simulink model "Excavator_Mevea_BucketDriveline"  (R2026a)
settings: Solver=ode23t  StopTime=29.5  FixedStep=1e-5  MaxStep=Ts  AbsTol=1e-3
PostLoadFcn:
  | set_param(bdroot,'IgnoredZcDiagnostic','none');
  | Excavator_Test_Scenario_Select('loadedBucketDigCycle');
  | Excavator_Mevea_params
StartFcn:
  | tic
StopFcn:
  | elapsedSimTime = toc;
  | disp(['Elapsed Sim Time = ' num2str(elapsedSimTime)]);
model workspace: external: MAT-File ExcavatorAssemblyDataStruct.mat (data not in the file)
undefined symbols (not defined in the file or in its folder): AToBRegOrificeVector, AToTOrificeVector, BiPOrificeVector, BoomC, boomHEArea, boomREArea, boomUpMaxQ, boomValve, BToTOrificeVector, BucketC, bucketCloseMaxQ, bucketOpenMaxQ, BucketR, bucketValve, DiscIntNeverNeededParam, fluids, gravity, K, Lambda, LeftBoomR, maxPumpDisp, minPumpDisp, nominalEngineSpeed, P28Assembly, PToAOrificeVector, PToBOrificeVector, pumpCmdNegRateLimit, pumpCmdPosRateLimit, RightBoomR, StickC, stickInMaxQ, stickOutMaxQ, StickR, stickValve, SwingC, swingDisplacement, swingHighSpeedThreshold, swingMaxQ, SwingR, swingSpeedQGain, swingValve, tau, valveCmdNegRateLimit, valveCmdPosRateLimit, X, x0, Y, Z
libraries: fl_lib x113, SimscapeFluids_lib x78, nesl_utility x61, sm_lib x55, simulink_extras x11, Excavator_Parts_Lib x6, sm_wheel_loader_lib x6, simulink x5, sdl_lib x4, SignalEditorBlockLib x1
(part 2 of 8)

== system Excavator_Mevea_BucketDriveline/Excavator/Hydraulics/RightPump ==
  Cmd : Inport
  Mechanical Rotational Reference : fl_lib/Mechanical/Rotational Elements/Mechanical Rotational Reference
  PS-Simulink Converter2 : nesl_utility/PS-Simulink Converter  PhysicalDomain=network_engine_domain  SubClassName=ps_output  LeftPortType=input  RightPortType=output  PseudoPeriodic=off  Frequencies=[]  VectorFormat=1-D array  Unit=bar  AffineConversion=off
  RightPump : SimscapeFluids_lib/Isothermal Liquid/Pumps & Motors/Variable-Displacement Pump (IL)  leakage_friction_spec=fluids.isothermal_liquid.pumps_motors.enum.pump_motor_loss_spec.input_efficiency  displacement_nominal=30 cm^3/rev  omega_nominal=188 rad/s  p_nominal=10 MPa  vol_eff_nominal=0.92  mech_eff_nominal=0.88  no_load_torque=0 N*m  p_diff_eff_TLU=[.1, 1, 2] MPa  omega_eff_TLU=[25, 50, 100, 200, 300, 400] rad/s  displacement_eff_TLU=[-30, -19, 19, 30] cm^3/rev  vol_eff_TLU=repmat([.816, .908, .954, .977, .981, .984; .325, .663, .831, .916, .925, .946; .137, .568, .78, .892, .893, .91], 1, 1, 4)  mech_eff_TLU=repmat([.996, .996, .996, .996, .996, .996; .988, .989, .989, .989, .989, .99; .981, .981, .982, .982, .983, .984], 1, 1, 4)  p_diff_loss_TLU=[.1, 1, 2] MPa  omega_loss_TLU=[25, 50, 100, 200, 300, 400] rad/s  displacement_loss_TLU=[-30, -19, 19, 30] cm^3/rev  vol_loss_TLU=repmat(1e-3 * [.023, .023, .023, .023, .0285, .032; .0844, .0842, .0845, .084, .1125, .108; .1079, .108, .11, .108, .1605, .18], 1, 1, 4) m^3/s  mech_loss_TLU=repmat([.002, .002, .002, .002, .002, .002; .0607, .0556, .0556, .0556, .0556, .0505; .1937, .1937, .1833, .1833, .1729, .1626], 1, 1, 4) N*m  vol_eff_min=1e-3  vol_eff_max=1  mech_eff_min=1e-3  mech_eff_max=1  pressure_threshold=1e-3 MPa  omega_threshold=10 rad/s  displacement_threshold=0.1 cm^3/rev  supplied_range_check=simscape.enum.assert.action.none  pump_mode_check=simscape.enum.assert.action.none  pressure_check=simscape.enum.assert.action.none  p_min_valid=0.101325 MPa
  RightPumpEM : fl_lib/Physical Signals/Sources/PS Constant  constant=1
  RightPumpEV : fl_lib/Physical Signals/Sources/PS Constant  constant=1
  RightPumpPrSensor : fl_lib/Isothermal Liquid/Sensors/Pressure Sensor (IL)  pressure_measure=foundation.enum.pressure_measure.gauge
  RightPumpVolChamber : fl_lib/Isothermal Liquid/Elements/Constant Volume Chamber (IL)  volume=pumpChamberVol mm^3  p_I_specify=on  p_I_priority=High  p_I=p0 bar  p_I_nominal_specify=off  p_I_nominal_value=1  p_I_nominal_unit=MPa
  Simulink-PS Converter1 : nesl_utility/Simulink-PS Converter  PhysicalDomain=network_engine_domain  SubClassName=ps_input  LeftPortType=input  RightPortType=output  PseudoPeriodic=off  Frequencies=[]  NoiseDistribution=none  NoiseParameters=[]  Unit=cm^3/rev  AffineConversion=off  FilteringAndDerivatives=provide  SimscapeFilterOrder=1  InputFilterTimeConstant=0.001  UdotUserProvided=0
  Transfer Fcn (with initial outputs) : simulink_extras/Additional Linear/Transfer Fcn (with initial outputs)  N=[1]  D="[0.01  1]"  Y0=p0  U0=p0
  R : PMIOPort  Side=Left
  A : PMIOPort  Port=2  Side=Left
  B : PMIOPort  Port=3  Side=Right
  p : Outport
  wires:
  PS-Simulink Converter2/1 -> Transfer Fcn (with initial outputs)/1
  Transfer Fcn (with initial outputs)/1 -> p/1
  Cmd/1 -> Simulink-PS Converter1/1
  connections:
  RightPumpEV/RConn1 -- RightPump/LConn2
  RightPumpPrSensor/RConn1 -- PS-Simulink Converter2/LConn1
  B/RConn1 -- RightPump/LConn4 -- RightPumpPrSensor/LConn1 -- RightPumpVolChamber/LConn1
  Simulink-PS Converter1/RConn1 -- RightPump/LConn1
  RightPumpEM/RConn1 -- RightPump/LConn3
  R/RConn1 -- RightPump/RConn1
  RightPump/RConn3 -- A/RConn1
  RightPump/RConn2 -- Mechanical Rotational Reference/LConn1

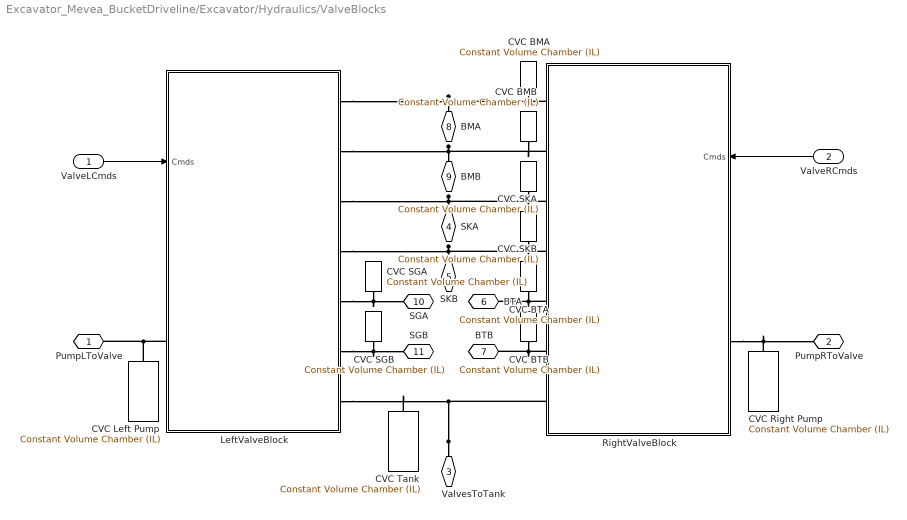
== system Excavator_Mevea_BucketDriveline/Excavator/Hydraulics/ValveBlocks ==
  ValveLCmds : Inport
  ValveRCmds : Inport  Port=2
  CVC BMA : fl_lib/Isothermal Liquid/Elements/Constant Volume Chamber (IL)  volume=vcVol m^3  p_I_specify=on  p_I_priority=High  p_I=initBoomHEPr bar  p_I_nominal_specify=off  p_I_nominal_value=1  p_I_nominal_unit=MPa
  CVC BMB : fl_lib/Isothermal Liquid/Elements/Constant Volume Chamber (IL)  volume=vcVol m^3  p_I_specify=on  p_I_priority=High  p_I=initBoomREPr bar  p_I_nominal_specify=off  p_I_nominal_value=1  p_I_nominal_unit=MPa
  CVC BTA : fl_lib/Isothermal Liquid/Elements/Constant Volume Chamber (IL)  volume=vcVol m^3  p_I_specify=on  p_I_priority=High  p_I=initBucketHEPr bar  p_I_nominal_specify=off  p_I_nominal_value=1  p_I_nominal_unit=MPa
  CVC BTB : fl_lib/Isothermal Liquid/Elements/Constant Volume Chamber (IL)  volume=vcVol m^3  p_I_specify=on  p_I_priority=High  p_I=initBucketREPr bar  p_I_nominal_specify=off  p_I_nominal_value=1  p_I_nominal_unit=MPa
  CVC Left Pump : fl_lib/Isothermal Liquid/Elements/Constant Volume Chamber (IL)  volume=vcVol m^3  p_I_specify=on  p_I_priority=High  p_I=p0 bar  p_I_nominal_specify=off  p_I_nominal_value=1  p_I_nominal_unit=MPa
  CVC Right Pump : fl_lib/Isothermal Liquid/Elements/Constant Volume Chamber (IL)  volume=vcVol m^3  p_I_specify=on  p_I_priority=High  p_I=p0 bar  p_I_nominal_specify=off  p_I_nominal_value=1  p_I_nominal_unit=MPa
  CVC SGA : fl_lib/Isothermal Liquid/Elements/Constant Volume Chamber (IL)  volume=vcVol m^3  p_I_specify=on  p_I_priority=High  p_I=initSwingAPr bar  p_I_nominal_specify=off  p_I_nominal_value=1  p_I_nominal_unit=MPa
  CVC SGB : fl_lib/Isothermal Liquid/Elements/Constant Volume Chamber (IL)  volume=vcVol m^3  p_I_specify=on  p_I_priority=High  p_I=initSwingBPr bar  p_I_nominal_specify=off  p_I_nominal_value=1  p_I_nominal_unit=MPa
  CVC SKA : fl_lib/Isothermal Liquid/Elements/Constant Volume Chamber (IL)  volume=vcVol m^3  p_I_specify=on  p_I_priority=High  p_I=initStickHEPr bar  p_I_nominal_specify=off  p_I_nominal_value=1  p_I_nominal_unit=MPa
  CVC SKB : fl_lib/Isothermal Liquid/Elements/Constant Volume Chamber (IL)  volume=vcVol m^3  p_I_specify=on  p_I_priority=High  p_I=initStickREPr bar  p_I_nominal_specify=off  p_I_nominal_value=1  p_I_nominal_unit=MPa
  CVC Tank : fl_lib/Isothermal Liquid/Elements/Constant Volume Chamber (IL)  volume=vcVol m^3  p_I_specify=off  p_I_priority=High  p_I=0.101325 MPa  p_I_nominal_specify=off  p_I_nominal_value=1  p_I_nominal_unit=MPa
  LeftValveBlock : Subsystem
      mask Display: image('Valve_Block_IMAGE.png');
  RightValveBlock : Subsystem
      settings: PortSchema="{\"entries\":[{\"content\":{\"sides\":[{\"content\":{\"connectorIds\":[\"LConn1\",\"LConn2\",\"LConn3\",\"LConn4\",\"LConn5\",\"LConn6\",\"LConn7\"]},\"type\":\"ConnectorPlacement.EquallySpacedRectSide\",\"uuid\":\"fd7eba1c-1e3a-4ec4-8a30-0aa9917de4dc\"},{\"content\":{\"connectorIds\":[\"In1\",\"RConn1\"],\"side\":\"RIGHT\"},\"type\":\"ConnectorPlacement.EquallySpacedRectSide\",\"uuid\":\"9d3cd55f-fb3f-4660-b4d9-215545d0bbbc\"},{\"content\":{\"connectorIds\":[],\"side\":\"TOP\"},\"type\":\"ConnectorPlacement.EquallySpacedRectSide\",\"uuid\":\"9eea4e27-675d-42da-a03e-9d9617f5a1f0\"}]},\"type\":\"ConnectorPlacement.EquallySpacedConnector\",\"uuid\":\"83287ec4-2b92-4936-b2f3-c04c41d999a3\"}],\"packageUris\":[\"http://schema.mathworks.com/mf0/Connector/R2020b\"],\"version\":\"1.0\"}"
      mask Display: image('Valve_Block_IMAGE.png');
  PumpLToValve : PMIOPort  Side=Left
  PumpRToValve : PMIOPort  Port=2  Side=Left
  ValvesToTank : PMIOPort  Port=3  Side=Left
  SKA : PMIOPort  Port=4  Side=Right
  SKB : PMIOPort  Port=5  Side=Right
  BTA : PMIOPort  Port=6  Side=Right
  BTB : PMIOPort  Port=7  Side=Right
  BMA : PMIOPort  Port=8  Side=Right
  BMB : PMIOPort  Port=9  Side=Right
  SGA : PMIOPort  Port=10  Side=Right
  SGB : PMIOPort  Port=11  Side=Right
  wires:
  ValveLCmds/1 -> LeftValveBlock/1(Cmds)
  ValveRCmds/1 -> RightValveBlock/1(Cmds)
  connections:
  RightValveBlock/LConn6 -- BTB/RConn1 -- CVC BTB/LConn1
  RightValveBlock/LConn5 -- BTA/RConn1 -- CVC BTA/LConn1
  LeftValveBlock/RConn6 -- CVC SGB/LConn1 -- SGB/RConn1
  LeftValveBlock/RConn5 -- CVC SGA/LConn1 -- SGA/RConn1
  BMA/RConn1 -- RightValveBlock/LConn1 -- CVC BMA/LConn1 -- LeftValveBlock/RConn1
  SKA/RConn1 -- RightValveBlock/LConn3 -- CVC SKA/LConn1 -- LeftValveBlock/RConn3
  BMB/RConn1 -- RightValveBlock/LConn2 -- CVC BMB/LConn1 -- LeftValveBlock/RConn2
  SKB/RConn1 -- RightValveBlock/LConn4 -- CVC SKB/LConn1 -- LeftValveBlock/RConn4
  RightValveBlock/RConn1 -- CVC Right Pump/LConn1 -- PumpRToValve/RConn1
  ValvesToTank/RConn1 -- CVC Tank/LConn1 -- LeftValveBlock/RConn7 -- RightValveBlock/LConn7
  LeftValveBlock/LConn1 -- CVC Left Pump/LConn1 -- PumpLToValve/RConn1

== system Excavator_Mevea_BucketDriveline/Excavator/Machine/BaseToChassis ==
  BaseToChassis : sm_lib/Joints/Revolute Joint  JointMode=Normal  CompositeWrenchDir=FollowerOnBase  CompositeWrenchFrame=BaseFrame  SenseConstraintForce=off  SenseConstraintTorque=off  SenseTotalForce=off  SenseTotalTorque=off  PositionTargetSpecify=on  PositionTargetPriority=High  PositionTargetValue=initSwingAngle  PositionTargetValueUnits=deg  VelocityTargetSpecify=on  VelocityTargetPriority=High  VelocityTargetValue=0  VelocityTargetValueUnits=deg/s  EquilibriumPosition=0  EquilibriumPositionUnits=deg  SpringStiffness=0  SpringStiffnessUnits=N*m/deg  DampingCoefficient=0  DampingCoefficientUnits=N*m/(deg/s)  LowerLimitSpecify=off  LowerLimitBound=-90  LowerLimitBoundUnits=deg  LowerLimitStiffness=1e4  LowerLimitStiffnessUnits=N*m/deg  LowerLimitDamping=10  LowerLimitDampingUnits=N*m/(deg/s)  LowerLimitTransitionRegionWidth=0.1  LowerLimitTransitionRegionWidthUnits=deg  UpperLimitSpecify=off  UpperLimitBound=90  UpperLimitBoundUnits=deg  UpperLimitStiffness=1e4  UpperLimitStiffnessUnits=N*m/deg  UpperLimitDamping=10  UpperLimitDampingUnits=N*m/(deg/s)  UpperLimitTransitionRegionWidth=0.1  UpperLimitTransitionRegionWidthUnits=deg  TorqueActuationMode=InputTorque  MotionActuationMode=ComputedMotion  SensePosition=off  SenseVelocity=on  SenseAcceleration=off  SenseTorqueForce=off  SenseLowerLimitTorqueForce=off  SenseUpperLimitTorqueForce=off
  PS-Simulink Converter : nesl_utility/PS-Simulink Converter  PhysicalDomain=network_engine_domain  SubClassName=ps_output  LeftPortType=input  RightPortType=output  PseudoPeriodic=off  Frequencies=[]  VectorFormat=inherit  Unit=rpm  AffineConversion=off
  Rotational Multibody Interface : fl_lib/Mechanical/Multibody Interfaces/Rotational Multibody Interface
  Simscape Bus : SimscapeBus  HierarchyStrings=SwingC;SwingR
  Transfer Fcn1 : TransferFcn  Denominator=[0.01 1]
  F : PMIOPort  Side=Right
  S : PMIOPort  Port=2  Side=Left
  B : PMIOPort  Port=3  Side=Left
  m : Outport
  wires:
  PS-Simulink Converter/1 -> Transfer Fcn1/1
  Transfer Fcn1/1 -> m/1
  connections:
  BaseToChassis/RConn1 -- F/RConn1
  Rotational Multibody Interface/RConn1 -- PS-Simulink Converter/LConn1 -- BaseToChassis/RConn2
  Rotational Multibody Interface/LConn1 -- BaseToChassis/LConn2
  Simscape Bus/RConn1 -- S/RConn1
  Simscape Bus/LConn1 -- Rotational Multibody Interface/LConn2
  Simscape Bus/LConn2 -- Rotational Multibody Interface/RConn2
  BaseToChassis/LConn1 -- B/RConn1

== system Excavator_Mevea_BucketDriveline/Excavator/Machine/Boom Cyl L ==
  BoomLeftCyl : Subsystem  Tag=4F70B330-6F24-E84C-8BE5-4F108E58AE93
  BoomLeftPiston : Subsystem  Tag=45215E48-B489-9D47-85FC-0A495393BD12
  BoomToLeftBoomPiston : sm_lib/Joints/Universal Joint  JointMode=Normal  CompositeWrenchDir=FollowerOnBase  CompositeWrenchFrame=BaseFrame  SenseConstraintForce=off  SenseConstraintTorque=off  SenseTotalForce=off  SenseTotalTorque=off  RxPositionTargetSpecify=off  RxPositionTargetPriority=High  RxPositionTargetValue=0  RxPositionTargetValueUnits=deg  RxVelocityTargetSpecify=off  RxVelocityTargetPriority=High  RxVelocityTargetValue=0  RxVelocityTargetValueUnits=deg/s  RxEquilibriumPosition=0  RxEquilibriumPositionUnits=deg  RxSpringStiffness=0  RxSpringStiffnessUnits=N*m/deg  RxDampingCoefficient=0  RxDampingCoefficientUnits=N*m/(deg/s)  RxLowerLimitSpecify=off  RxLowerLimitBound=-90  RxLowerLimitBoundUnits=deg  RxLowerLimitStiffness=1e4  RxLowerLimitStiffnessUnits=N*m/deg  RxLowerLimitDamping=10  RxLowerLimitDampingUnits=N*m/(deg/s)  RxLowerLimitTransitionRegionWidth=0.1  RxLowerLimitTransitionRegionWidthUnits=deg  RxUpperLimitSpecify=off  RxUpperLimitBound=90  RxUpperLimitBoundUnits=deg  RxUpperLimitStiffness=1e4  RxUpperLimitStiffnessUnits=N*m/deg  RxUpperLimitDamping=10  RxUpperLimitDampingUnits=N*m/(deg/s)  RxUpperLimitTransitionRegionWidth=0.1  RxUpperLimitTransitionRegionWidthUnits=deg  RxTorqueActuationMode=NoTorque  RxMotionActuationMode=ComputedMotion  RxSensePosition=off  RxSenseVelocity=off  RxSenseAcceleration=off  RxSenseTorqueForce=off  RxSenseLowerLimitTorqueForce=off  RxSenseUpperLimitTorqueForce=off  RyPositionTargetSpecify=off  RyPositionTargetPriority=High  RyPositionTargetValue=0  RyPositionTargetValueUnits=deg  RyVelocityTargetSpecify=off  RyVelocityTargetPriority=High  RyVelocityTargetValue=0  RyVelocityTargetValueUnits=deg/s  RyEquilibriumPosition=0  RyEquilibriumPositionUnits=deg  RySpringStiffness=0  RySpringStiffnessUnits=N*m/deg  RyDampingCoefficient=0  RyDampingCoefficientUnits=N*m/(deg/s)  RyLowerLimitSpecify=off  RyLowerLimitBound=-90  RyLowerLimitBoundUnits=deg  RyLowerLimitStiffness=1e4  RyLowerLimitStiffnessUnits=N*m/deg  RyLowerLimitDamping=10  RyLowerLimitDampingUnits=N*m/(deg/s)  RyLowerLimitTransitionRegionWidth=0.1  RyLowerLimitTransitionRegionWidthUnits=deg  RyUpperLimitSpecify=off  RyUpperLimitBound=90  RyUpperLimitBoundUnits=deg  RyUpperLimitStiffness=1e4  RyUpperLimitStiffnessUnits=N*m/deg  RyUpperLimitDamping=10  RyUpperLimitDampingUnits=N*m/(deg/s)  RyUpperLimitTransitionRegionWidth=0.1  RyUpperLimitTransitionRegionWidthUnits=deg  RyTorqueActuationMode=NoTorque  RyMotionActuationMode=ComputedMotion  RySensePosition=off  RySenseVelocity=off  RySenseAcceleration=off  RySenseTorqueForce=off  RySenseLowerLimitTorqueForce=off  RySenseUpperLimitTorqueForce=off
  ChassisToLeftBoomCyl : sm_lib/Joints/Universal Joint  JointMode=Normal  CompositeWrenchDir=FollowerOnBase  CompositeWrenchFrame=BaseFrame  SenseConstraintForce=off  SenseConstraintTorque=off  SenseTotalForce=off  SenseTotalTorque=off  RxPositionTargetSpecify=off  RxPositionTargetPriority=High  RxPositionTargetValue=0  RxPositionTargetValueUnits=deg  RxVelocityTargetSpecify=off  RxVelocityTargetPriority=High  RxVelocityTargetValue=0  RxVelocityTargetValueUnits=deg/s  RxEquilibriumPosition=0  RxEquilibriumPositionUnits=deg  RxSpringStiffness=0  RxSpringStiffnessUnits=N*m/deg  RxDampingCoefficient=0  RxDampingCoefficientUnits=N*m/(deg/s)  RxLowerLimitSpecify=off  RxLowerLimitBound=-90  RxLowerLimitBoundUnits=deg  RxLowerLimitStiffness=1e4  RxLowerLimitStiffnessUnits=N*m/deg  RxLowerLimitDamping=10  RxLowerLimitDampingUnits=N*m/(deg/s)  RxLowerLimitTransitionRegionWidth=0.1  RxLowerLimitTransitionRegionWidthUnits=deg  RxUpperLimitSpecify=off  RxUpperLimitBound=90  RxUpperLimitBoundUnits=deg  RxUpperLimitStiffness=1e4  RxUpperLimitStiffnessUnits=N*m/deg  RxUpperLimitDamping=10  RxUpperLimitDampingUnits=N*m/(deg/s)  RxUpperLimitTransitionRegionWidth=0.1  RxUpperLimitTransitionRegionWidthUnits=deg  RxTorqueActuationMode=NoTorque  RxMotionActuationMode=ComputedMotion  RxSensePosition=off  RxSenseVelocity=off  RxSenseAcceleration=off  RxSenseTorqueForce=off  RxSenseLowerLimitTorqueForce=off  RxSenseUpperLimitTorqueForce=off  RyPositionTargetSpecify=off  RyPositionTargetPriority=High  RyPositionTargetValue=0  RyPositionTargetValueUnits=deg  RyVelocityTargetSpecify=off  RyVelocityTargetPriority=High  RyVelocityTargetValue=0  RyVelocityTargetValueUnits=deg/s  RyEquilibriumPosition=0  RyEquilibriumPositionUnits=deg  RySpringStiffness=0  RySpringStiffnessUnits=N*m/deg  RyDampingCoefficient=0  RyDampingCoefficientUnits=N*m/(deg/s)  RyLowerLimitSpecify=off  RyLowerLimitBound=-90  RyLowerLimitBoundUnits=deg  RyLowerLimitStiffness=1e4  RyLowerLimitStiffnessUnits=N*m/deg  RyLowerLimitDamping=10  RyLowerLimitDampingUnits=N*m/(deg/s)  RyLowerLimitTransitionRegionWidth=0.1  RyLowerLimitTransitionRegionWidthUnits=deg  RyUpperLimitSpecify=off  RyUpperLimitBound=90  RyUpperLimitBoundUnits=deg  RyUpperLimitStiffness=1e4  RyUpperLimitStiffnessUnits=N*m/deg  RyUpperLimitDamping=10  RyUpperLimitDampingUnits=N*m/(deg/s)  RyUpperLimitTransitionRegionWidth=0.1  RyUpperLimitTransitionRegionWidthUnits=deg  RyTorqueActuationMode=NoTorque  RyMotionActuationMode=ComputedMotion  RySensePosition=off  RySenseVelocity=off  RySenseAcceleration=off  RySenseTorqueForce=off  RySenseLowerLimitTorqueForce=off  RySenseUpperLimitTorqueForce=off
  LeftBoomCylToLeftBoomPiston : Subsystem  Tag=020d177e-0dad-473d-ac20-6fcc1e17d1fc
  m : PMIOPort  Side=Right
  Act : PMIOPort  Port=2  Side=Left
  B : PMIOPort  Port=3  Side=Left
  F : PMIOPort  Port=4  Side=Right
  connections:
  BoomToLeftBoomPiston/LConn1 -- F/RConn1
  ChassisToLeftBoomCyl/RConn1 -- BoomLeftCyl/LConn1
  Act/RConn1 -- m/RConn1 -- LeftBoomCylToLeftBoomPiston/LConn2
  BoomToLeftBoomPiston/RConn1 -- BoomLeftPiston/RConn1
  BoomLeftCyl/RConn1 -- LeftBoomCylToLeftBoomPiston/LConn1
  B/RConn1 -- ChassisToLeftBoomCyl/LConn1
  LeftBoomCylToLeftBoomPiston/RConn1 -- BoomLeftPiston/LConn1

== system Excavator_Mevea_BucketDriveline/Excavator/Machine/Boom Cyl R ==
  BoomRightCyl : Subsystem  Tag=807666EC-A6D7-8B4A-99F9-B3248F920B99
  BoomRightPiston : Subsystem  Tag=00EE293A-0F1A-9247-9056-19EF67FE5161
  BoomToRightBoomPiston : sm_lib/Joints/Universal Joint  JointMode=Normal  CompositeWrenchDir=FollowerOnBase  CompositeWrenchFrame=BaseFrame  SenseConstraintForce=off  SenseConstraintTorque=off  SenseTotalForce=off  SenseTotalTorque=off  RxPositionTargetSpecify=off  RxPositionTargetPriority=High  RxPositionTargetValue=0  RxPositionTargetValueUnits=deg  RxVelocityTargetSpecify=off  RxVelocityTargetPriority=High  RxVelocityTargetValue=0  RxVelocityTargetValueUnits=deg/s  RxEquilibriumPosition=0  RxEquilibriumPositionUnits=deg  RxSpringStiffness=0  RxSpringStiffnessUnits=N*m/deg  RxDampingCoefficient=0  RxDampingCoefficientUnits=N*m/(deg/s)  RxLowerLimitSpecify=off  RxLowerLimitBound=-90  RxLowerLimitBoundUnits=deg  RxLowerLimitStiffness=1e4  RxLowerLimitStiffnessUnits=N*m/deg  RxLowerLimitDamping=10  RxLowerLimitDampingUnits=N*m/(deg/s)  RxLowerLimitTransitionRegionWidth=0.1  RxLowerLimitTransitionRegionWidthUnits=deg  RxUpperLimitSpecify=off  RxUpperLimitBound=90  RxUpperLimitBoundUnits=deg  RxUpperLimitStiffness=1e4  RxUpperLimitStiffnessUnits=N*m/deg  RxUpperLimitDamping=10  RxUpperLimitDampingUnits=N*m/(deg/s)  RxUpperLimitTransitionRegionWidth=0.1  RxUpperLimitTransitionRegionWidthUnits=deg  RxTorqueActuationMode=NoTorque  RxMotionActuationMode=ComputedMotion  RxSensePosition=off  RxSenseVelocity=off  RxSenseAcceleration=off  RxSenseTorqueForce=off  RxSenseLowerLimitTorqueForce=off  RxSenseUpperLimitTorqueForce=off  RyPositionTargetSpecify=off  RyPositionTargetPriority=High  RyPositionTargetValue=0  RyPositionTargetValueUnits=deg  RyVelocityTargetSpecify=off  RyVelocityTargetPriority=High  RyVelocityTargetValue=0  RyVelocityTargetValueUnits=deg/s  RyEquilibriumPosition=0  RyEquilibriumPositionUnits=deg  RySpringStiffness=0  RySpringStiffnessUnits=N*m/deg  RyDampingCoefficient=0  RyDampingCoefficientUnits=N*m/(deg/s)  RyLowerLimitSpecify=off  RyLowerLimitBound=-90  RyLowerLimitBoundUnits=deg  RyLowerLimitStiffness=1e4  RyLowerLimitStiffnessUnits=N*m/deg  RyLowerLimitDamping=10  RyLowerLimitDampingUnits=N*m/(deg/s)  RyLowerLimitTransitionRegionWidth=0.1  RyLowerLimitTransitionRegionWidthUnits=deg  RyUpperLimitSpecify=off  RyUpperLimitBound=90  RyUpperLimitBoundUnits=deg  RyUpperLimitStiffness=1e4  RyUpperLimitStiffnessUnits=N*m/deg  RyUpperLimitDamping=10  RyUpperLimitDampingUnits=N*m/(deg/s)  RyUpperLimitTransitionRegionWidth=0.1  RyUpperLimitTransitionRegionWidthUnits=deg  RyTorqueActuationMode=NoTorque  RyMotionActuationMode=ComputedMotion  RySensePosition=off  RySenseVelocity=off  RySenseAcceleration=off  RySenseTorqueForce=off  RySenseLowerLimitTorqueForce=off  RySenseUpperLimitTorqueForce=off
  ChassisToRightBoomCyl : sm_lib/Joints/Universal Joint  JointMode=Normal  CompositeWrenchDir=FollowerOnBase  CompositeWrenchFrame=BaseFrame  SenseConstraintForce=off  SenseConstraintTorque=off  SenseTotalForce=off  SenseTotalTorque=off  RxPositionTargetSpecify=off  RxPositionTargetPriority=High  RxPositionTargetValue=0  RxPositionTargetValueUnits=deg  RxVelocityTargetSpecify=off  RxVelocityTargetPriority=High  RxVelocityTargetValue=0  RxVelocityTargetValueUnits=deg/s  RxEquilibriumPosition=0  RxEquilibriumPositionUnits=deg  RxSpringStiffness=0  RxSpringStiffnessUnits=N*m/deg  RxDampingCoefficient=0  RxDampingCoefficientUnits=N*m/(deg/s)  RxLowerLimitSpecify=off  RxLowerLimitBound=-90  RxLowerLimitBoundUnits=deg  RxLowerLimitStiffness=1e4  RxLowerLimitStiffnessUnits=N*m/deg  RxLowerLimitDamping=10  RxLowerLimitDampingUnits=N*m/(deg/s)  RxLowerLimitTransitionRegionWidth=0.1  RxLowerLimitTransitionRegionWidthUnits=deg  RxUpperLimitSpecify=off  RxUpperLimitBound=90  RxUpperLimitBoundUnits=deg  RxUpperLimitStiffness=1e4  RxUpperLimitStiffnessUnits=N*m/deg  RxUpperLimitDamping=10  RxUpperLimitDampingUnits=N*m/(deg/s)  RxUpperLimitTransitionRegionWidth=0.1  RxUpperLimitTransitionRegionWidthUnits=deg  RxTorqueActuationMode=NoTorque  RxMotionActuationMode=ComputedMotion  RxSensePosition=off  RxSenseVelocity=off  RxSenseAcceleration=off  RxSenseTorqueForce=off  RxSenseLowerLimitTorqueForce=off  RxSenseUpperLimitTorqueForce=off  RyPositionTargetSpecify=off  RyPositionTargetPriority=High  RyPositionTargetValue=0  RyPositionTargetValueUnits=deg  RyVelocityTargetSpecify=off  RyVelocityTargetPriority=High  RyVelocityTargetValue=0  RyVelocityTargetValueUnits=deg/s  RyEquilibriumPosition=0  RyEquilibriumPositionUnits=deg  RySpringStiffness=0  RySpringStiffnessUnits=N*m/deg  RyDampingCoefficient=0  RyDampingCoefficientUnits=N*m/(deg/s)  RyLowerLimitSpecify=off  RyLowerLimitBound=-90  RyLowerLimitBoundUnits=deg  RyLowerLimitStiffness=1e4  RyLowerLimitStiffnessUnits=N*m/deg  RyLowerLimitDamping=10  RyLowerLimitDampingUnits=N*m/(deg/s)  RyLowerLimitTransitionRegionWidth=0.1  RyLowerLimitTransitionRegionWidthUnits=deg  RyUpperLimitSpecify=off  RyUpperLimitBound=90  RyUpperLimitBoundUnits=deg  RyUpperLimitStiffness=1e4  RyUpperLimitStiffnessUnits=N*m/deg  RyUpperLimitDamping=10  RyUpperLimitDampingUnits=N*m/(deg/s)  RyUpperLimitTransitionRegionWidth=0.1  RyUpperLimitTransitionRegionWidthUnits=deg  RyTorqueActuationMode=NoTorque  RyMotionActuationMode=ComputedMotion  RySensePosition=off  RySenseVelocity=off  RySenseAcceleration=off  RySenseTorqueForce=off  RySenseLowerLimitTorqueForce=off  RySenseUpperLimitTorqueForce=off
  RightBoomCylToRightBoomPiston : Subsystem  Tag=f4b02144-fc21-4459-875a-429d4adb33c6
  m : PMIOPort  Side=Right
  F : PMIOPort  Port=2  Side=Right
  Act : PMIOPort  Port=3  Side=Left
  B : PMIOPort  Port=4  Side=Left
  connections:
  ChassisToRightBoomCyl/LConn1 -- B/RConn1
  BoomToRightBoomPiston/RConn1 -- BoomRightPiston/RConn1
  RightBoomCylToRightBoomPiston/RConn1 -- BoomRightPiston/LConn1
  BoomRightCyl/LConn1 -- ChassisToRightBoomCyl/RConn1
  BoomRightCyl/RConn1 -- RightBoomCylToRightBoomPiston/LConn2
  Act/RConn1 -- RightBoomCylToRightBoomPiston/LConn1
  BoomToRightBoomPiston/LConn1 -- F/RConn1

== system Excavator_Mevea_BucketDriveline/Excavator/Machine/Bucket Cyl ==
  BucketCyl : Subsystem  Tag=9FAF18D5-1596-3A48-9F24-977D2E18A318
  BucketCylToBucketPiston : Subsystem  Tag=47fb7853-569f-437e-8d3d-7cddda445dda
  BucketPiston : Subsystem  Tag=EF45ED1F-ED8A-8D4B-830B-367867E4E96A
  BucketPistonToBucketLink : sm_lib/Joints/Universal Joint  JointMode=Normal  CompositeWrenchDir=FollowerOnBase  CompositeWrenchFrame=BaseFrame  SenseConstraintForce=off  SenseConstraintTorque=off  SenseTotalForce=off  SenseTotalTorque=off  RxPositionTargetSpecify=off  RxPositionTargetPriority=High  RxPositionTargetValue=0  RxPositionTargetValueUnits=deg  RxVelocityTargetSpecify=off  RxVelocityTargetPriority=High  RxVelocityTargetValue=0  RxVelocityTargetValueUnits=deg/s  RxEquilibriumPosition=0  RxEquilibriumPositionUnits=deg  RxSpringStiffness=0  RxSpringStiffnessUnits=N*m/deg  RxDampingCoefficient=0  RxDampingCoefficientUnits=N*m/(deg/s)  RxLowerLimitSpecify=off  RxLowerLimitBound=-90  RxLowerLimitBoundUnits=deg  RxLowerLimitStiffness=1e4  RxLowerLimitStiffnessUnits=N*m/deg  RxLowerLimitDamping=10  RxLowerLimitDampingUnits=N*m/(deg/s)  RxLowerLimitTransitionRegionWidth=0.1  RxLowerLimitTransitionRegionWidthUnits=deg  RxUpperLimitSpecify=off  RxUpperLimitBound=90  RxUpperLimitBoundUnits=deg  RxUpperLimitStiffness=1e4  RxUpperLimitStiffnessUnits=N*m/deg  RxUpperLimitDamping=10  RxUpperLimitDampingUnits=N*m/(deg/s)  RxUpperLimitTransitionRegionWidth=0.1  RxUpperLimitTransitionRegionWidthUnits=deg  RxTorqueActuationMode=NoTorque  RxMotionActuationMode=ComputedMotion  RxSensePosition=off  RxSenseVelocity=off  RxSenseAcceleration=off  RxSenseTorqueForce=off  RxSenseLowerLimitTorqueForce=off  RxSenseUpperLimitTorqueForce=off  RyPositionTargetSpecify=off  RyPositionTargetPriority=High  RyPositionTargetValue=0  RyPositionTargetValueUnits=deg  RyVelocityTargetSpecify=off  RyVelocityTargetPriority=High  RyVelocityTargetValue=0  RyVelocityTargetValueUnits=deg/s  RyEquilibriumPosition=0  RyEquilibriumPositionUnits=deg  RySpringStiffness=0  RySpringStiffnessUnits=N*m/deg  RyDampingCoefficient=0  RyDampingCoefficientUnits=N*m/(deg/s)  RyLowerLimitSpecify=off  RyLowerLimitBound=-90  RyLowerLimitBoundUnits=deg  RyLowerLimitStiffness=1e4  RyLowerLimitStiffnessUnits=N*m/deg  RyLowerLimitDamping=10  RyLowerLimitDampingUnits=N*m/(deg/s)  RyLowerLimitTransitionRegionWidth=0.1  RyLowerLimitTransitionRegionWidthUnits=deg  RyUpperLimitSpecify=off  RyUpperLimitBound=90  RyUpperLimitBoundUnits=deg  RyUpperLimitStiffness=1e4  RyUpperLimitStiffnessUnits=N*m/deg  RyUpperLimitDamping=10  RyUpperLimitDampingUnits=N*m/(deg/s)  RyUpperLimitTransitionRegionWidth=0.1  RyUpperLimitTransitionRegionWidthUnits=deg  RyTorqueActuationMode=NoTorque  RyMotionActuationMode=ComputedMotion  RySensePosition=off  RySenseVelocity=off  RySenseAcceleration=off  RySenseTorqueForce=off  RySenseLowerLimitTorqueForce=off  RySenseUpperLimitTorqueForce=off
  StickToBucketCyl : sm_lib/Joints/Universal Joint  JointMode=Normal  CompositeWrenchDir=FollowerOnBase  CompositeWrenchFrame=BaseFrame  SenseConstraintForce=off  SenseConstraintTorque=off  SenseTotalForce=off  SenseTotalTorque=off  RxPositionTargetSpecify=off  RxPositionTargetPriority=High  RxPositionTargetValue=0  RxPositionTargetValueUnits=deg  RxVelocityTargetSpecify=off  RxVelocityTargetPriority=High  RxVelocityTargetValue=0  RxVelocityTargetValueUnits=deg/s  RxEquilibriumPosition=0  RxEquilibriumPositionUnits=deg  RxSpringStiffness=0  RxSpringStiffnessUnits=N*m/deg  RxDampingCoefficient=0  RxDampingCoefficientUnits=N*m/(deg/s)  RxLowerLimitSpecify=off  RxLowerLimitBound=-90  RxLowerLimitBoundUnits=deg  RxLowerLimitStiffness=1e4  RxLowerLimitStiffnessUnits=N*m/deg  RxLowerLimitDamping=10  RxLowerLimitDampingUnits=N*m/(deg/s)  RxLowerLimitTransitionRegionWidth=0.1  RxLowerLimitTransitionRegionWidthUnits=deg  RxUpperLimitSpecify=off  RxUpperLimitBound=90  RxUpperLimitBoundUnits=deg  RxUpperLimitStiffness=1e4  RxUpperLimitStiffnessUnits=N*m/deg  RxUpperLimitDamping=10  RxUpperLimitDampingUnits=N*m/(deg/s)  RxUpperLimitTransitionRegionWidth=0.1  RxUpperLimitTransitionRegionWidthUnits=deg  RxTorqueActuationMode=NoTorque  RxMotionActuationMode=ComputedMotion  RxSensePosition=off  RxSenseVelocity=off  RxSenseAcceleration=off  RxSenseTorqueForce=off  RxSenseLowerLimitTorqueForce=off  RxSenseUpperLimitTorqueForce=off  RyPositionTargetSpecify=off  RyPositionTargetPriority=High  RyPositionTargetValue=0  RyPositionTargetValueUnits=deg  RyVelocityTargetSpecify=off  RyVelocityTargetPriority=High  RyVelocityTargetValue=0  RyVelocityTargetValueUnits=deg/s  RyEquilibriumPosition=0  RyEquilibriumPositionUnits=deg  RySpringStiffness=0  RySpringStiffnessUnits=N*m/deg  RyDampingCoefficient=0  RyDampingCoefficientUnits=N*m/(deg/s)  RyLowerLimitSpecify=off  RyLowerLimitBound=-90  RyLowerLimitBoundUnits=deg  RyLowerLimitStiffness=1e4  RyLowerLimitStiffnessUnits=N*m/deg  RyLowerLimitDamping=10  RyLowerLimitDampingUnits=N*m/(deg/s)  RyLowerLimitTransitionRegionWidth=0.1  RyLowerLimitTransitionRegionWidthUnits=deg  RyUpperLimitSpecify=off  RyUpperLimitBound=90  RyUpperLimitBoundUnits=deg  RyUpperLimitStiffness=1e4  RyUpperLimitStiffnessUnits=N*m/deg  RyUpperLimitDamping=10  RyUpperLimitDampingUnits=N*m/(deg/s)  RyUpperLimitTransitionRegionWidth=0.1  RyUpperLimitTransitionRegionWidthUnits=deg  RyTorqueActuationMode=NoTorque  RyMotionActuationMode=ComputedMotion  RySensePosition=off  RySenseVelocity=off  RySenseAcceleration=off  RySenseTorqueForce=off  RySenseLowerLimitTorqueForce=off  RySenseUpperLimitTorqueForce=off
  m : PMIOPort  Side=Right
  Act : PMIOPort  Port=2  Side=Left
  B : PMIOPort  Port=3  Side=Left
  F : PMIOPort  Port=4  Side=Right
  connections:
  BucketPistonToBucketLink/LConn1 -- BucketPiston/RConn1
  BucketCylToBucketPiston/RConn1 -- BucketPiston/LConn1
  StickToBucketCyl/RConn1 -- BucketCyl/LConn1
  BucketPistonToBucketLink/RConn1 -- F/RConn1
  BucketCyl/RConn1 -- BucketCylToBucketPiston/LConn1
  B/RConn1 -- StickToBucketCyl/LConn1
  Act/RConn1 -- m/RConn1 -- BucketCylToBucketPiston/LConn2

== system Excavator_Mevea_BucketDriveline/Excavator/Machine/Gravity ==
  Constant : Constant  Value=0
  Constant1 : Constant  Value=0
  Constant2 : Constant  Value=gravity
  Integrator : Integrator  LimitOutput=on  UpperSaturationLimit=0  LowerSaturationLimit=gravity
  Mux : Mux  Inputs=3
  g : Outport
  wires:
  Constant1/1 -> Mux/1
  Integrator/1 -> Mux/3
  Constant/1 -> Mux/2
  Constant2/1 -> Integrator/1
  Mux/1 -> g/1

== system Excavator_Mevea_BucketDriveline/Excavator/Machine/Ground ==
  Mevea Soil : sm_lib/Body Elements/File Solid  ExtGeomFileName=DesolateOutbackProjectionTarget.stl  UnitType=Custom  ExtGeomFileUnits=m  StepReaderType=HEX  ExportConvexHullGeometry=off  InertiaType=CalculateFromGeometry  BasedOnType=Mass  Density=1000  DensityUnits=kg/m^3  Mass=1  MassUnits=kg  CenterOfMass=[0 0 0]  CenterOfMassUnits=m  MomentsOfInertia=[1 1 1]  MomentsOfInertiaUnits=kg*m^2  ProductsOfInertia=[0 0 0]  ProductsOfInertiaUnits=kg*m^2  GraphicType=FromGeometry  MarkerShape=Sphere  MarkerSize=10  GraphicVisPropType=SimpleVisualProperties  GraphicDiffuseColor=[1 0.9333 0.5098]  GraphicOpacity=1  GraphicSpecularColor=[0.5 0.5 0.5 1.0]  GraphicAmbientColor=[0.15 0.15 0.15 1.0]  GraphicEmissiveColor=[0.0 0.0 0.0 1.0]  GraphicShininess=75  DoExposeReferenceFrame=on  SerializedFrames=<Frames/>
  Transform MeveaSoil : sm_lib/Frames and Transforms/Rigid Transform  RotationMethod=AlignedAxes  FollAlignAxisA=+Z  BaseAlignAxisA=+X  FollAlignAxisB=+Y  BaseAlignAxisB=+Z  RotationStandardAxis=+Z  RotationAngle=0.0  RotationAngleUnits=deg  RotationArbitraryAxis=[0 0 1]  RotationSequenceAxes=FollowerAxes  RotationSequence=XYX  RotationSequenceAngles=[0 0 0]  RotationSequenceAnglesUnits=deg  RotationMatrix=[1 0 0; 0 1 0; 0 0 1]  Quaternion=[1 0 0 0]  TranslationMethod=Cartesian  TranslationCartesianOffset=[130 60 -1.02]  TranslationCartesianOffsetUnits=m  TranslationStandardAxis=+Z  TranslationStandardOffset=0  TranslationStandardOffsetUnits=m  TranslationROffset=0  TranslationROffsetUnits=m  TranslationThetaOffset=0  TranslationThetaOffsetUnits=deg  TranslationZOffset=0  TranslationZOffsetUnits=m
  W : PMIOPort  Side=Left
  connections:
  Transform MeveaSoil/LConn1 -- W/RConn1
  Mevea Soil/RConn1 -- Transform MeveaSoil/RConn1

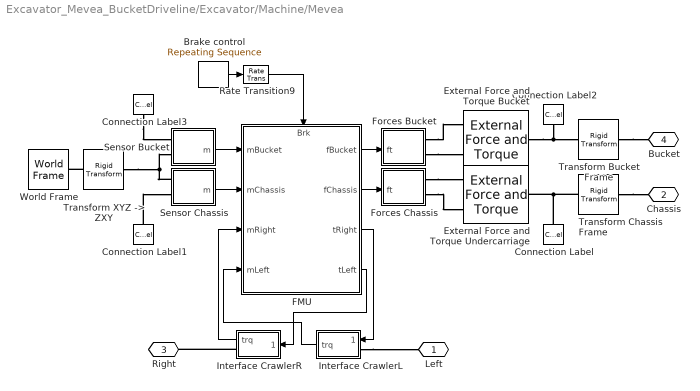
== system Excavator_Mevea_BucketDriveline/Excavator/Machine/Mevea ==
  Brake control : simulink/Sources/Repeating Sequence  rep_seq_t=[0 10 11 15 40]  rep_seq_y=[0 0 1e3 3e4 3e4]
  Connection Label : ConnectionLabel  Label=FrCha
  Connection Label1 : ConnectionLabel  Label=FrCha
  Connection Label2 : ConnectionLabel  Label=FrBkt
  Connection Label3 : ConnectionLabel  Label=FrBkt
  External Force and Torque Bucket : sm_lib/Forces and Torques/External Force and Torque  EnableForceX=off  EnableForceY=off  EnableForceZ=off  EnableForce=on  ForceResolutionFrame=World  EnableTorqueX=off  EnableTorqueY=off  EnableTorqueZ=off  EnableTorque=on  TorqueResolutionFrame=World
  External Force and Torque Undercarriage : sm_lib/Forces and Torques/External Force and Torque  EnableForceX=off  EnableForceY=off  EnableForceZ=off  EnableForce=on  ForceResolutionFrame=World  EnableTorqueX=off  EnableTorqueY=off  EnableTorqueZ=off  EnableTorque=on  TorqueResolutionFrame=World
  FMU : Subsystem
      settings: PortSchema="{\"entries\":[{\"content\":{\"sides\":[{\"content\":{\"connectorIds\":[\"In1\",\"In2\",\"In3\",\"In4\"]},\"type\":\"ConnectorPlacement.EquallySpacedRectSide\",\"uuid\":\"055b99ae-8ba1-4879-96e6-ed4e2bbe2bd3\"},{\"content\":{\"connectorIds\":[\"Out1\",\"Out2\",\"Out3\",\"Out4\"],\"side\":\"RIGHT\"},\"type\":\"ConnectorPlacement.EquallySpacedRectSide\",\"uuid\":\"8ef5c778-b1fb-41f7-b691-6635c4b0e749\"},{\"content\":{\"connectorIds\":[\"In5\"],\"side\":\"TOP\"},\"type\":\"ConnectorPlacement.EquallySpacedRectSide\",\"uuid\":\"e5d2bdf0-51e6-4bbe-a7af-8a5026cd1e42\"},{\"content\":{\"side\":\"BOTTOM\"},\"type\":\"ConnectorPlacement.EquallySpacedRectSide\",\"uuid\":\"db0503a6-333f-48db-aa4c-d4d077da243e\"}]},\"type\":\"ConnectorPlacement.EquallySpacedConnector\",\"uuid\":\"a6e99301-9c57-41f4-8ce8-405dbecb781c\"}],\"packageUris\":[\"http://schema.mathworks.com/mf0/Connector/R2020b\"],\"version\":\"1.0\"}"
  Forces Bucket : Subsystem
  Forces Chassis : Subsystem
  Interface CrawlerL : Subsystem
  Interface CrawlerR : Subsystem
  Rate Transition9 : RateTransition  OutPortSampleTime=mbsTimeStep
  Sensor Bucket : Subsystem
  Sensor Chassis : Subsystem
  Transform Bucket Frame : sm_lib/Frames and Transforms/Rigid Transform  RotationMethod=StandardAxis  FollAlignAxisA=+X  BaseAlignAxisA=+Y  FollAlignAxisB=+Y  BaseAlignAxisB=+Z  RotationStandardAxis=+Z  RotationAngle=148.94  RotationAngleUnits=deg  RotationArbitraryAxis=[0 0 1]  RotationSequenceAxes=FollowerAxes  RotationSequence=XYX  RotationSequenceAngles=[0 0 0]  RotationSequenceAnglesUnits=deg  RotationMatrix=[1 0 0;0 1 0;0 0 1]  Quaternion=[1 0 0 0]  TranslationMethod=None  TranslationCartesianOffset=[0 0 0]  TranslationCartesianOffsetUnits=m  TranslationStandardAxis=+Z  TranslationStandardOffset=0  TranslationStandardOffsetUnits=m  TranslationROffset=0  TranslationROffsetUnits=m  TranslationThetaOffset=0  TranslationThetaOffsetUnits=deg  TranslationZOffset=0  TranslationZOffsetUnits=m
  Transform Chassis Frame : sm_lib/Frames and Transforms/Rigid Transform  RotationMethod=AlignedAxes  FollAlignAxisA=+Z  BaseAlignAxisA=+X  FollAlignAxisB=+Y  BaseAlignAxisB=+Z  RotationStandardAxis=+Z  RotationAngle=0  RotationAngleUnits=deg  RotationArbitraryAxis=[0 0 1]  RotationSequenceAxes=FollowerAxes  RotationSequence=XYX  RotationSequenceAngles=[0 0 0]  RotationSequenceAnglesUnits=deg  RotationMatrix=[1 0 0;0 1 0;0 0 1]  Quaternion=[1 0 0 0]  TranslationMethod=None  TranslationCartesianOffset=[0 0 0]  TranslationCartesianOffsetUnits=m  TranslationStandardAxis=+Z  TranslationStandardOffset=0  TranslationStandardOffsetUnits=m  TranslationROffset=0  TranslationROffsetUnits=m  TranslationThetaOffset=0  TranslationThetaOffsetUnits=deg  TranslationZOffset=0  TranslationZOffsetUnits=m
  "Transform XYZ -> ZXY" : sm_lib/Frames and Transforms/Rigid Transform  RotationMethod=AlignedAxes  FollAlignAxisA=+Z  BaseAlignAxisA=+X  FollAlignAxisB=+Y  BaseAlignAxisB=+Z  RotationStandardAxis=+Z  RotationAngle=0  RotationAngleUnits=deg  RotationArbitraryAxis=[0 0 1]  RotationSequenceAxes=FollowerAxes  RotationSequence=XYX  RotationSequenceAngles=[0 0 0]  RotationSequenceAnglesUnits=deg  RotationMatrix=[1 0 0;0 1 0;0 0 1]  Quaternion=[1 0 0 0]  TranslationMethod=None  TranslationCartesianOffset=[0 0 0]  TranslationCartesianOffsetUnits=m  TranslationStandardAxis=+Z  TranslationStandardOffset=0  TranslationStandardOffsetUnits=m  TranslationROffset=0  TranslationROffsetUnits=m  TranslationThetaOffset=0  TranslationThetaOffsetUnits=deg  TranslationZOffset=0  TranslationZOffsetUnits=m
  World Frame : sm_lib/Frames and Transforms/World Frame
  Left : PMIOPort  Side=Left
  Chassis : PMIOPort  Port=2  Side=Left
  Right : PMIOPort  Port=3  Side=Right
  Bucket : PMIOPort  Port=4  Side=Right
  wires:
  Brake control/1 -> Rate Transition9/1
  Sensor Bucket/1(m) -> FMU/1(mBucket)
  Sensor Chassis/1(m) -> FMU/2(mChassis)
  Rate Transition9/1 -> FMU/5(Brk)
  Interface CrawlerR/1(trq) -> FMU/3(mRight)
  Interface CrawlerL/1(trq) -> FMU/4(mLeft)
  FMU/3(tRight) -> Interface CrawlerL/1(spd)
  FMU/4(tLeft) -> Interface CrawlerR/1(spd)
  FMU/2(fChassis) -> Forces Chassis/1(ft)
  FMU/1(fBucket) -> Forces Bucket/1(ft)
  connections:
  "Transform XYZ -> ZXY"/LConn1 -- World Frame/RConn1
  Interface CrawlerL/LConn1 -- Left/RConn1
  Transform Bucket Frame/LConn1 -- Bucket/RConn1
  Transform Chassis Frame/LConn1 -- Chassis/RConn1
  Interface CrawlerR/RConn1 -- Right/RConn1
  External Force and Torque Bucket/RConn1 -- Connection Label2/LConn1 -- Transform Bucket Frame/RConn1
  "Transform XYZ -> ZXY"/RConn1 -- Sensor Bucket/LConn2 -- Sensor Chassis/LConn1
  Transform Chassis Frame/RConn1 -- External Force and Torque Undercarriage/RConn1 -- Connection Label/LConn1
  Forces Bucket/RConn1 -- External Force and Torque Bucket/LConn1
  Forces Bucket/RConn2 -- External Force and Torque Bucket/LConn2
  Forces Chassis/RConn1 -- External Force and Torque Undercarriage/LConn1
  Forces Chassis/RConn2 -- External Force and Torque Undercarriage/LConn2
  Connection Label1/LConn1 -- Sensor Chassis/LConn2
  Connection Label3/LConn1 -- Sensor Bucket/LConn1

== system Excavator_Mevea_BucketDriveline/Excavator/Machine/Pos CG ==
  Bus Creator : BusCreator  Inputs=2
  PS-Simulink Converter : nesl_utility/PS-Simulink Converter  PhysicalDomain=network_engine_domain  SubClassName=ps_output  LeftPortType=input  RightPortType=output  PseudoPeriodic=off  Frequencies=[]  VectorFormat=inherit  Unit=inherit  AffineConversion=off
  PS-Simulink Converter1 : nesl_utility/PS-Simulink Converter  PhysicalDomain=network_engine_domain  SubClassName=ps_output  LeftPortType=input  RightPortType=output  PseudoPeriodic=off  Frequencies=[]  VectorFormat=inherit  Unit=inherit  AffineConversion=off
  Terminator : Terminator
  Transform Sensor : sm_lib/Frames and Transforms/Transform Sensor  MeasurementFrame=Base  RotationSequence=XYX  SenseAngle=off  SenseAxis=off  SenseQ=off  SenseR=off  SenseRotationSequence=off  SenseOmegaX=off  SenseOmegaY=off  SenseOmegaZ=off  SenseOmega=off  SenseQDot=off  SenseRDot=off  SenseRotationSequenceDot=off  SenseAlphaX=off  SenseAlphaY=off  SenseAlphaZ=off  SenseAlpha=off  SenseQDDot=off  SenseRDDot=off  SenseX=off  SenseY=on  SenseZ=on  SenseXYZ=off  SenseRad=off  SenseAzim=off  SenseDist=off  SenseInc=off  SenseXDot=off  SenseYDot=off  SenseZDot=off  SenseXYZDot=off  SenseRadDot=off  SenseAzimDot=off  SenseDistDot=off  SenseIncDot=off  SenseXDDot=off  SenseYDDot=off  SenseZDDot=off  SenseXYZDDot=off  SenseRadDDot=off  SenseAzimDDot=off  SenseDistDDot=off  SenseIncDDot=off
  F : PMIOPort  Side=Right
  B : PMIOPort  Port=2  Side=Left
  wires:
  Bus Creator/1 -> Terminator/1  "Bucket_CG"
  PS-Simulink Converter/1 -> Bus Creator/1  "xLong"
  PS-Simulink Converter1/1 -> Bus Creator/2  "xVert"
  connections:
  PS-Simulink Converter1/LConn1 -- Transform Sensor/RConn3
  Transform Sensor/LConn1 -- B/RConn1
  Transform Sensor/RConn2 -- PS-Simulink Converter/LConn1
  Transform Sensor/RConn1 -- F/RConn1

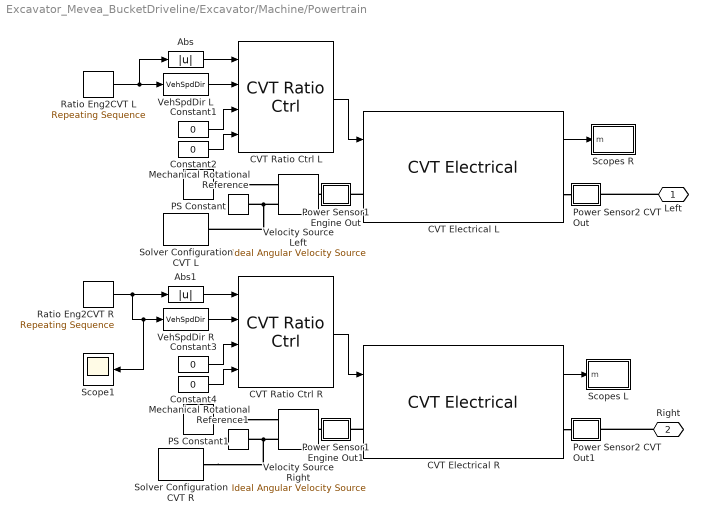
== system Excavator_Mevea_BucketDriveline/Excavator/Machine/Powertrain ==
  Abs : Abs  ZeroCross=off  SaturateOnIntegerOverflow=off
  Abs1 : Abs  ZeroCross=off  SaturateOnIntegerOverflow=off
  CVT Electrical L : sm_wheel_loader_lib/CVT Electrical  VariantControl=Electrical
  CVT Electrical R : sm_wheel_loader_lib/CVT Electrical  VariantControl=Electrical
  CVT Ratio Ctrl L : sm_wheel_loader_lib/Controller/CVT Ratio Ctrl  SystemSampleTime=-1  VariantActivationTime=update diagram  EmptyChoice=off  PassThrough=off  PassThroughVariantControl=(default)  EmptyChoiceVariantControl=(default)  AllowFlexibleInterface=on  Latency=0  AutoFrameSizeCalculation=off
  CVT Ratio Ctrl R : sm_wheel_loader_lib/Controller/CVT Ratio Ctrl  SystemSampleTime=-1  VariantActivationTime=update diagram  EmptyChoice=off  PassThrough=off  PassThroughVariantControl=(default)  EmptyChoiceVariantControl=(default)  AllowFlexibleInterface=on  Latency=0  AutoFrameSizeCalculation=off
  Constant{1..4} (4 alike) : Constant  Value=0
  Mechanical Rotational Reference : fl_lib/Mechanical/Rotational Elements/Mechanical Rotational Reference
  Mechanical Rotational Reference1 : fl_lib/Mechanical/Rotational Elements/Mechanical Rotational Reference
  PS Constant : fl_lib/Physical Signals/Sources/PS Constant  constant=2200 rpm
  PS Constant1 : fl_lib/Physical Signals/Sources/PS Constant  constant=2200 rpm
  Power Sensor1 Engine Out : Subsystem
  Power Sensor1 Engine Out1 : Subsystem
  Power Sensor2 CVT Out : Subsystem
  Power Sensor2 CVT Out1 : Subsystem
  Ratio Eng2CVT L : simulink/Sources/Repeating Sequence  rep_seq_t=[0 1.5 4.5 6.5 8 10 11 40]  rep_seq_y=[0 0 0.08 0.08 0.05 0.01 0 0]
  Ratio Eng2CVT R : simulink/Sources/Repeating Sequence  rep_seq_t=[0 1.5 4.5 6.5 8 10 11 40]  rep_seq_y=[0 0 0.08 0.08 0.05 0.01 0 0]
  Scope1 : Scope
      settings: ActiveDisplayYMinimum=-0.01  ActiveDisplayYMaximum=0.09
  Scopes L : Subsystem
  Scopes R : Subsystem
  Solver Configuration CVT L : nesl_utility/Solver Configuration  PhysicalDomain=network_engine_domain  SubClassName=solver  LeftPortType=input  RightPortType=generic  Tones=[]  Harmonics=[]  SimulateNoise=off  Profile=off  UseLocalSampling=off  EnableSwitchedLinearOptims=on  FrequencyDomain=off  UseCCode=off  RelTol=0.001  AbsTol=1e-06  MinStep=1e-09  ToWorkspace=off  RevertToSquareIcSolve=off  NumHomotopyIterations=100  PhasorMode=off  PhasorModeNumHarmonics=1  ConsistencySolver=NEWTON_XTOL_AFTER_FTOL  CanonicalOrdering=UNORDERED  OptimizeIntermediates=UNOPTIMIZED  IndexReductionMethod=DerivativeReplacement  DoDC=off  ResidualTolerance=1e-09  ConsistencyTolSource=GLOBAL  ConsistencyAbsTol=0.001  ConsistencyRelTol=0.001  ConsistencyTolFactor=0.001  UseLocalSolver=off  LocalSolverChoice=NE_BACKWARD_EULER_ADVANCER  ResolveIndetEquations=on  FunctionEvalNumThread=1  LocalSolverSampleTime=0.001  DoFixedCost=off  MaxNonlinIter=1  MaxModeIter=2  ComputeImpulses=off  ImpulseIterations=2  LinearAlgebra=Sparse  LinearAlgebraNumThread=0  EquationFormulation=NE_TIME_EF  DelaysMemoryBudget=1024  AutomaticFiltering=on  FilteringTimeConstant=0.001  PartitionStorageMethod=AS_NEEDED  PartitionMemoryBudget=1024  PartitionMethod=FAST  MultibodyUseLocalSolver=off  MultibodyLocalSolverChoice=ODE1  MultibodyLocalSolverSampleTime=0.001
  Solver Configuration CVT R : nesl_utility/Solver Configuration  PhysicalDomain=network_engine_domain  SubClassName=solver  LeftPortType=input  RightPortType=generic  Tones=[]  Harmonics=[]  SimulateNoise=off  Profile=off  UseLocalSampling=off  EnableSwitchedLinearOptims=on  FrequencyDomain=off  UseCCode=off  RelTol=0.001  AbsTol=1e-06  MinStep=1e-09  ToWorkspace=off  RevertToSquareIcSolve=off  NumHomotopyIterations=100  PhasorMode=off  PhasorModeNumHarmonics=1  ConsistencySolver=NEWTON_XTOL_AFTER_FTOL  CanonicalOrdering=UNORDERED  OptimizeIntermediates=UNOPTIMIZED  IndexReductionMethod=DerivativeReplacement  DoDC=off  ResidualTolerance=1e-09  ConsistencyTolSource=GLOBAL  ConsistencyAbsTol=0.001  ConsistencyRelTol=0.001  ConsistencyTolFactor=0.001  UseLocalSolver=off  LocalSolverChoice=NE_BACKWARD_EULER_ADVANCER  ResolveIndetEquations=on  FunctionEvalNumThread=1  LocalSolverSampleTime=0.001  DoFixedCost=off  MaxNonlinIter=1  MaxModeIter=2  ComputeImpulses=off  ImpulseIterations=2  LinearAlgebra=Sparse  LinearAlgebraNumThread=0  EquationFormulation=NE_TIME_EF  DelaysMemoryBudget=1024  AutomaticFiltering=on  FilteringTimeConstant=0.001  PartitionStorageMethod=AS_NEEDED  PartitionMemoryBudget=1024  PartitionMethod=FAST  MultibodyUseLocalSolver=off  MultibodyLocalSolverChoice=ODE1  MultibodyLocalSolverSampleTime=0.001
  VehSpdDir L : sm_wheel_loader_lib/Controller/Desired Ratio Calc/VehSpdDir  SystemSampleTime=-1  VariantActivationTime=update diagram  EmptyChoice=off  PassThrough=off  PassThroughVariantControl=(default)  EmptyChoiceVariantControl=(default)  AllowFlexibleInterface=on  Latency=0  AutoFrameSizeCalculation=off
  VehSpdDir R : sm_wheel_loader_lib/Controller/Desired Ratio Calc/VehSpdDir  SystemSampleTime=-1  VariantActivationTime=update diagram  EmptyChoice=off  PassThrough=off  PassThroughVariantControl=(default)  EmptyChoiceVariantControl=(default)  AllowFlexibleInterface=on  Latency=0  AutoFrameSizeCalculation=off
  Velocity Source Left : fl_lib/Mechanical/Mechanical Sources/Ideal Angular Velocity Source
  Velocity Source Right : fl_lib/Mechanical/Mechanical Sources/Ideal Angular Velocity Source
  Left : PMIOPort  Side=Left
  Right : PMIOPort  Port=2  Side=Right
  wires:
  Abs/1 -> CVT Ratio Ctrl L/1
  Ratio Eng2CVT R/1 -> Scope1/1, VehSpdDir R/1, Abs1/1
  CVT Ratio Ctrl R/1 -> CVT Electrical R/1
  Abs1/1 -> CVT Ratio Ctrl R/1
  CVT Ratio Ctrl L/1 -> CVT Electrical L/1
  VehSpdDir L/1 -> CVT Ratio Ctrl L/2
  Constant1/1 -> CVT Ratio Ctrl L/3
  VehSpdDir R/1 -> CVT Ratio Ctrl R/2
  CVT Electrical L/1 -> Scopes R/1(m)
  Ratio Eng2CVT L/1 -> VehSpdDir L/1, Abs/1
  Constant2/1 -> CVT Ratio Ctrl L/4
  Constant4/1 -> CVT Ratio Ctrl R/4
  Constant3/1 -> CVT Ratio Ctrl R/3
  CVT Electrical R/1 -> Scopes L/1(m)
  connections:
  Power Sensor1 Engine Out1/LConn1 -- Velocity Source Right/LConn1
  Mechanical Rotational Reference/LConn1 -- Solver Configuration CVT L/RConn1 -- Velocity Source Left/RConn2
  CVT Electrical R/RConn1 -- Power Sensor2 CVT Out1/LConn1
  Solver Configuration CVT R/RConn1 -- Mechanical Rotational Reference1/LConn1 -- Velocity Source Right/RConn2
  CVT Electrical R/LConn1 -- Power Sensor1 Engine Out1/RConn1
  PS Constant/RConn1 -- Velocity Source Left/RConn1
  CVT Electrical L/RConn1 -- Power Sensor2 CVT Out/LConn1
  CVT Electrical L/LConn1 -- Power Sensor1 Engine Out/RConn1
  PS Constant1/RConn1 -- Velocity Source Right/RConn1
  Power Sensor1 Engine Out/LConn1 -- Velocity Source Left/LConn1
  Left/RConn1 -- Power Sensor2 CVT Out/RConn1
  Right/RConn1 -- Power Sensor2 CVT Out1/RConn1
